simulink model "BenchMark"  (R2016b)
settings: Solver=VariableStepAuto  StartTime=0.0  StopTime=10.0  RelTol=1e-3
settings Model: Creator=Mojtaba  LastModifiedBy=Mojtaba

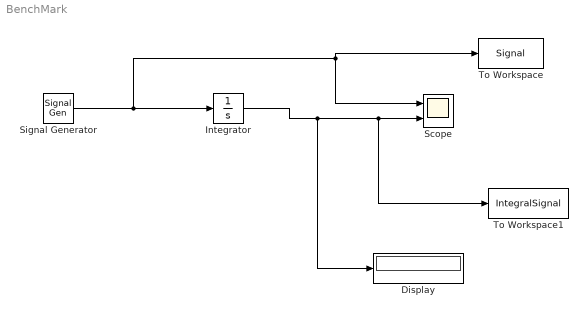
== system BenchMark ==
  Display : Display
  Integrator : Integrator
  Scope : Scope  NumInputPorts=2
  Signal Generator : SignalGenerator  Amplitude=20
  To Workspace : ToWorkspace  VariableName=Signal  SaveFormat=Timeseries  SampleTime=-1
  To Workspace1 : ToWorkspace  VariableName=IntegralSignal  SaveFormat=Timeseries  SampleTime=-1
  wires:
  Signal Generator/1 -> Scope/1, To Workspace/1, Integrator/1
  Integrator/1 -> Display/1, To Workspace1/1, Scope/2
